simulink model "satcomv2"  (R2024b)
settings: Solver=VariableStepAuto  StartTime=0.0  StopTime=10.0  RelTol=1e-3
settings Model: Creator=user  LastModifiedBy=user

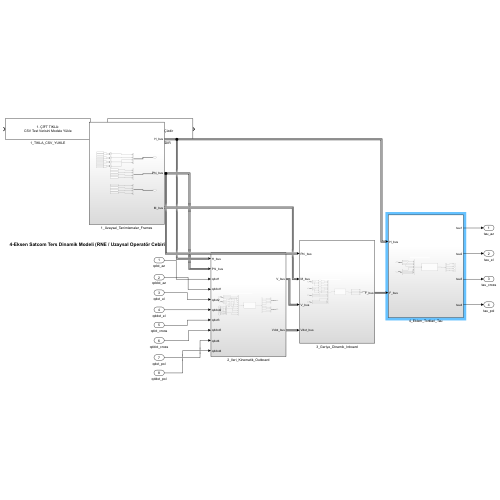
[thumbnail: Simulink's stored preview of the top-level diagram]
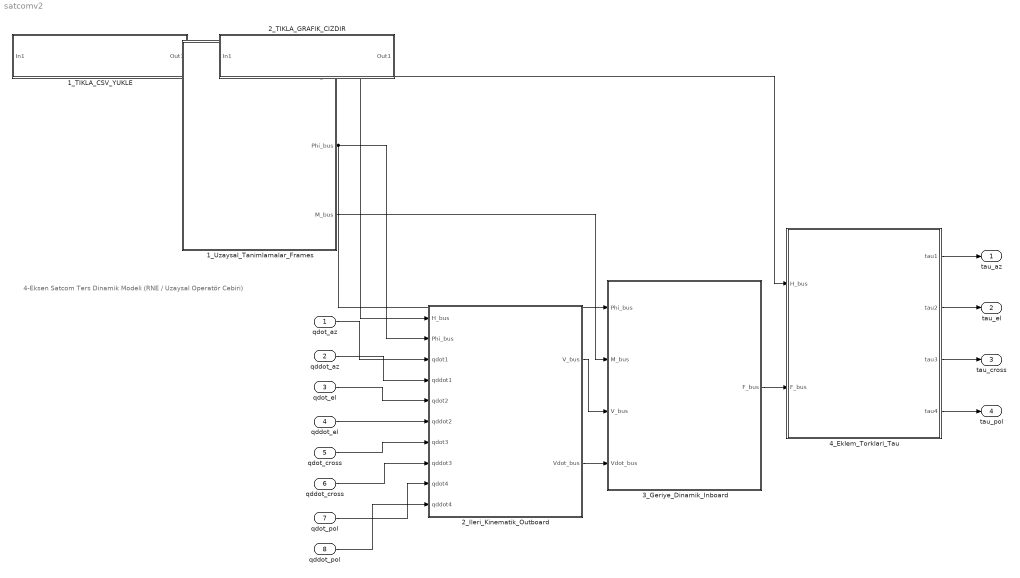
== system satcomv2 ==
  note: 4-Eksen Satcom Ters Dinamik Modeli (RNE / Uzaysal Operatör Cebiri)
  qdot_az : Inport
  qddot_az : Inport  Port=2
  qdot_el : Inport  Port=3
  qddot_el : Inport  Port=4
  qdot_cross : Inport  Port=5
  qddot_cross : Inport  Port=6
  qdot_pol : Inport  Port=7
  qddot_pol : Inport  Port=8
  1_TIKLA_CSV_YUKLE : Subsystem
      settings: OpenFcn=[f,p]=uigetfile({'*.csv;*.xlsx'}); if f~=0, mat=readmatrix(fullfile(p,f)); t=mat(:,2); t=t(:); v=mat(:,5); v=v(:); a=mat(:,7); a=a(:); % Sürücüden gelen akım (veya count) bilgisini Kt sabiti ile % çarparak motorun ürettiği gerçek Torka (Nm) dönüştürüyoruz.tau_real=mat(:,9) * 1.41; tau_real=tau_real(:); z=zeros(size(t)); assignin('base','in_qdot_az',timeseries(v,t)); assignin('base','in_qddot_az',timeseries(a,t)); assignin('base','in_zero',timeseries(z,t)); assignin('base','csv_zaman',t); assignin('base','csv_tork',tau_real); set_param(bdroot,'LoadExternalInput','on'); set_param(bdroot,'ExternalInput','in_qdot_az, in_qddot_az, in_zero, in_zero, in_zero, in_zero, in_zero, in_zero'); set_param(bdroot,'StopTime',num2str(t(end))); msgbox('Test Verileri Yüklendi! Sürücü çıkışı Kt=1.41 sabitiyle Nm cinsine dönüştürüldü.','BAŞARILI'); end
      mask Display: disp('1. ÇİFT TIKLA:\nCSV Test Verisini Modele Yükle');
  1_Uzaysal_Tanimlamalar_Frames : Subsystem
  2_Ileri_Kinematik_Outboard : Subsystem
  2_TIKLA_GRAFIK_CIZDIR : Subsystem
      settings: OpenFcn=try, simOut = evalin('base', 'out'); tau_raw = double(simOut.yout{1}.Values.Data(:)); t_sim = double(simOut.yout{1}.Values.Time(:)); [t_u, idx] = unique(t_sim); tau_u = tau_raw(idx); zaman = evalin('base', 'csv_zaman'); zaman = zaman(:); tau_real = evalin('base', 'csv_tork'); tau_real = tau_real(:); tau_model = interp1(t_u, tau_u, zaman, 'linear', 'extrap'); tau_model = tau_model(:); figure('Name', 'Saf Dinamik Model vs Gerçek Test', 'NumberTitle', 'off'); plot(zaman, tau_model, 'b', 'LineWidth', 1.5); hold on; plot(zaman, tau_real, 'r--', 'LineWidth', 1.2); title('Azimut Motoru - Tork İhtiyacı (Fiziksel Model vs Sürücü Çıkışı)'); xlabel('Zaman (s)'); ylabel('Tork (Nm)'); legend('Model Üretilen Tork (RNE İdeal Fiziği)', 'CSV İçindeki Gerçek Tork (Kt=1.41)'); grid on; SonucTablosu = table(zaman, tau_model, tau_real, 'VariableNames', {'Zaman_saniye', 'Model_Uretilen_Tork_Nm', 'Gercek_Sistem_Tork_Referansi'}); writetable(SonucTablosu, 'Model_Tork_Sonuclari.csv'); disp('Doğrulama verileri Model_Tork_Sonuclari.csv olarak başarıyla kaydedildi!'); catch ME, errordlg(sprintf('GRAFİK ÇİZİLEMEDİ!\\n\\nHata:\\n%s\\n\\nLütfen simülasyonu çalıştırdığınızdan (RUN) emin olun.', ME.message), 'Sistem Hatası'); end
      mask Display: disp('2. ÇİFT TIKLA:\nSaf Model Tork Grafiğini Çizdir');
  3_Geriye_Dinamik_Inboard : Subsystem
  4_Eklem_Torklari_Tau : Subsystem
  tau_az : Outport
  tau_el : Outport  Port=2
  tau_cross : Outport  Port=3
  tau_pol : Outport  Port=4
  wires:
  qddot_az/1 -> 2_Ileri_Kinematik_Outboard/4(qddot1)
  1_Uzaysal_Tanimlamalar_Frames/1(H_bus) -> 4_Eklem_Torklari_Tau/1(H_bus), 2_Ileri_Kinematik_Outboard/1(H_bus)
  1_Uzaysal_Tanimlamalar_Frames/2(Phi_bus) -> 3_Geriye_Dinamik_Inboard/1(Phi_bus), 2_Ileri_Kinematik_Outboard/2(Phi_bus)
  1_Uzaysal_Tanimlamalar_Frames/3(M_bus) -> 3_Geriye_Dinamik_Inboard/2(M_bus)
  qdot_az/1 -> 2_Ileri_Kinematik_Outboard/3(qdot1)
  qdot_el/1 -> 2_Ileri_Kinematik_Outboard/5(qdot2)
  qddot_el/1 -> 2_Ileri_Kinematik_Outboard/6(qddot2)
  qdot_cross/1 -> 2_Ileri_Kinematik_Outboard/7(qdot3)
  qddot_cross/1 -> 2_Ileri_Kinematik_Outboard/8(qddot3)
  qdot_pol/1 -> 2_Ileri_Kinematik_Outboard/9(qdot4)
  qddot_pol/1 -> 2_Ileri_Kinematik_Outboard/10(qddot4)
  2_Ileri_Kinematik_Outboard/1(V_bus) -> 3_Geriye_Dinamik_Inboard/3(V_bus)
  2_Ileri_Kinematik_Outboard/2(Vdot_bus) -> 3_Geriye_Dinamik_Inboard/4(Vdot_bus)
  3_Geriye_Dinamik_Inboard/1(F_bus) -> 4_Eklem_Torklari_Tau/2(F_bus)
  4_Eklem_Torklari_Tau/1(tau1) -> tau_az/1
  4_Eklem_Torklari_Tau/2(tau2) -> tau_el/1
  4_Eklem_Torklari_Tau/3(tau3) -> tau_cross/1
  4_Eklem_Torklari_Tau/4(tau4) -> tau_pol/1

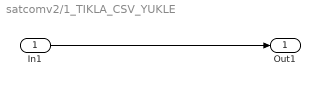
== system satcomv2/1_TIKLA_CSV_YUKLE ==
  In1 : Inport
  Out1 : Outport
  wires:
  In1/1 -> Out1/1

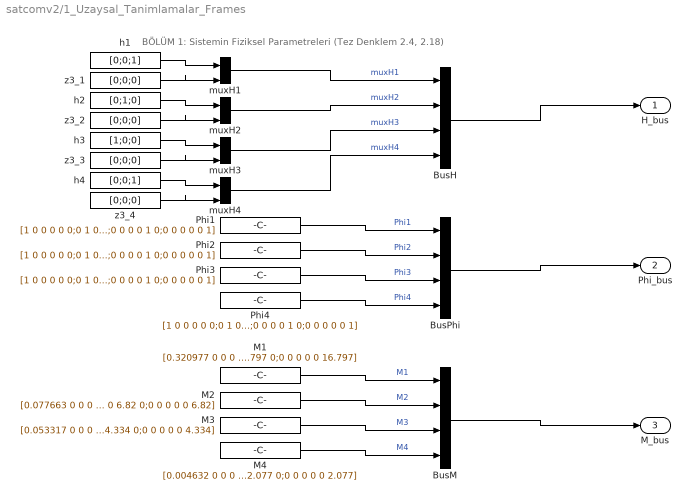
== system satcomv2/1_Uzaysal_Tanimlamalar_Frames ==
  note: BÖLÜM 1: Sistemin Fiziksel Parametreleri (Tez Denklem 2.4, 2.18)
  BusH : BusCreator  Inputs=4
  BusM : BusCreator  Inputs=4
  BusPhi : BusCreator  Inputs=4
  M1 : Constant  Value=[0.320977 0 0 0 0 0;0 0.320977 0 0 0 0;0 0 0.320977 0 0 0;0 0 0 16.797 0 0;0 0 0 0 16.797 0;0 0 0 0 0 16.797]
  M2 : Constant  Value=[0.077663 0 0 0 0 0;0 0.077663 0 0 0 0;0 0 0.077663 0 0 0;0 0 0 6.82 0 0;0 0 0 0 6.82 0;0 0 0 0 0 6.82]
  M3 : Constant  Value=[0.053317 0 0 0 0 0;0 0.053317 0 0 0 0;0 0 0.053317 0 0 0;0 0 0 4.334 0 0;0 0 0 0 4.334 0;0 0 0 0 0 4.334]
  M4 : Constant  Value=[0.004632 0 0 0 0 0;0 0.004632 0 0 0 0;0 0 0.004632 0 0 0;0 0 0 2.077 0 0;0 0 0 0 2.077 0;0 0 0 0 0 2.077]
  Phi{1..4} (4 alike) : Constant  Value=[1 0 0 0 0 0;0 1 0 0 0 0;0 0 1 0 0 0;0 0 0 1 0 0;0 0 0 0 1 0;0 0 0 0 0 1]
  h1 : Constant  Value=[0;0;1]
  h2 : Constant  Value=[0;1;0]
  h3 : Constant  Value=[1;0;0]
  h4 : Constant  Value=[0;0;1]
  muxH{1..4} (4 alike) : Mux  Inputs=2
  z3_{1..4} (4 alike) : Constant  Value=[0;0;0]
  H_bus : Outport
  Phi_bus : Outport  Port=2
  M_bus : Outport  Port=3
  wires:
  h1/1 -> muxH1/1
  z3_1/1 -> muxH1/2
  muxH1/1 -> BusH/1  "muxH1"
  h2/1 -> muxH2/1
  z3_2/1 -> muxH2/2
  muxH2/1 -> BusH/2  "muxH2"
  h3/1 -> muxH3/1
  z3_3/1 -> muxH3/2
  muxH3/1 -> BusH/3  "muxH3"
  h4/1 -> muxH4/1
  z3_4/1 -> muxH4/2
  muxH4/1 -> BusH/4  "muxH4"
  BusH/1 -> H_bus/1
  Phi1/1 -> BusPhi/1  "Phi1"
  Phi2/1 -> BusPhi/2  "Phi2"
  Phi3/1 -> BusPhi/3  "Phi3"
  Phi4/1 -> BusPhi/4  "Phi4"
  BusPhi/1 -> Phi_bus/1
  M1/1 -> BusM/1  "M1"
  M2/1 -> BusM/2  "M2"
  M3/1 -> BusM/3  "M3"
  M4/1 -> BusM/4  "M4"
  BusM/1 -> M_bus/1

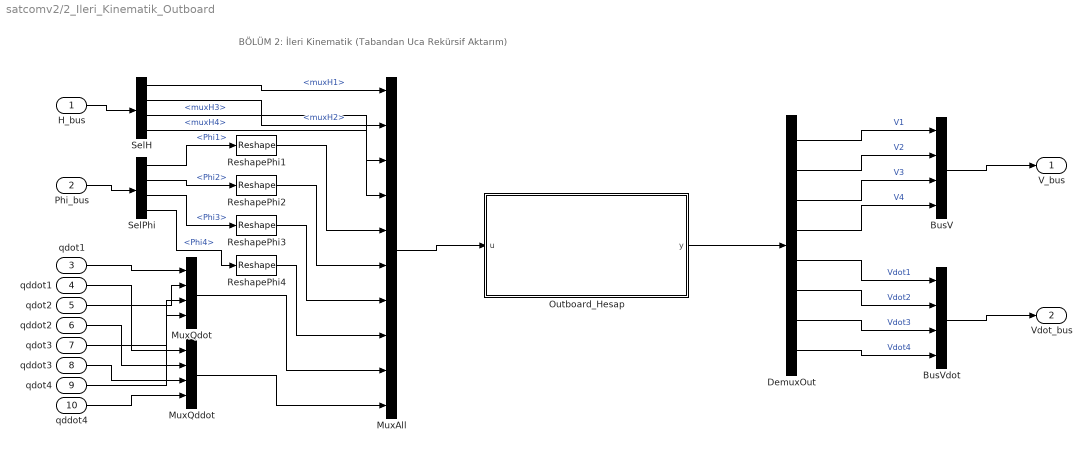
== system satcomv2/2_Ileri_Kinematik_Outboard ==
  note: BÖLÜM 2: İleri Kinematik (Tabandan Uca Rekürsif Aktarım)
  H_bus : Inport
  Phi_bus : Inport  Port=2
  qdot1 : Inport  Port=3
  qddot1 : Inport  Port=4
  qdot2 : Inport  Port=5
  qddot2 : Inport  Port=6
  qdot3 : Inport  Port=7
  qddot3 : Inport  Port=8
  qdot4 : Inport  Port=9
  qddot4 : Inport  Port=10
  BusV : BusCreator  Inputs=4
  BusVdot : BusCreator  Inputs=4
  DemuxOut : Demux  Outputs=[6 6 6 6 6 6 6 6]
  MuxAll : Mux  Inputs=10
  MuxQddot : Mux
  MuxQdot : Mux
  Outboard_Hesap : MATLAB Function  TreatAsAtomicUnit=on
  ReshapePhi{1..4} (4 alike) : Reshape
  SelH : BusSelector  OutputSignals=muxH1,muxH2,muxH3,muxH4
  SelPhi : BusSelector  OutputSignals=Phi1,Phi2,Phi3,Phi4
  V_bus : Outport
  Vdot_bus : Outport  Port=2
  wires:
  H_bus/1 -> SelH/1
  Phi_bus/1 -> SelPhi/1
  qdot1/1 -> MuxQdot/1
  qddot1/1 -> MuxQddot/1
  qdot2/1 -> MuxQdot/2
  qddot2/1 -> MuxQddot/2
  qdot3/1 -> MuxQdot/3
  qddot3/1 -> MuxQddot/3
  qdot4/1 -> MuxQdot/4
  qddot4/1 -> MuxQddot/4
  SelH/1 -> MuxAll/1  "<muxH1>"
  SelPhi/1 -> ReshapePhi1/1  "<Phi1>"
  ReshapePhi1/1 -> MuxAll/5
  SelH/2 -> MuxAll/2  "<muxH2>"
  SelPhi/2 -> ReshapePhi2/1  "<Phi2>"
  ReshapePhi2/1 -> MuxAll/6
  SelH/3 -> MuxAll/3  "<muxH3>"
  SelPhi/3 -> ReshapePhi3/1  "<Phi3>"
  ReshapePhi3/1 -> MuxAll/7
  SelH/4 -> MuxAll/4  "<muxH4>"
  SelPhi/4 -> ReshapePhi4/1  "<Phi4>"
  ReshapePhi4/1 -> MuxAll/8
  MuxQdot/1 -> MuxAll/9
  MuxQddot/1 -> MuxAll/10
  MuxAll/1 -> Outboard_Hesap/1(u)
  Outboard_Hesap/1(y) -> DemuxOut/1
  DemuxOut/1 -> BusV/1  "V1"
  DemuxOut/5 -> BusVdot/1  "Vdot1"
  DemuxOut/2 -> BusV/2  "V2"
  DemuxOut/6 -> BusVdot/2  "Vdot2"
  DemuxOut/3 -> BusV/3  "V3"
  DemuxOut/7 -> BusVdot/3  "Vdot3"
  DemuxOut/4 -> BusV/4  "V4"
  DemuxOut/8 -> BusVdot/4  "Vdot4"
  BusV/1 -> V_bus/1
  BusVdot/1 -> Vdot_bus/1

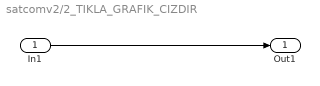
== system satcomv2/2_TIKLA_GRAFIK_CIZDIR ==
  In1 : Inport
  Out1 : Outport
  wires:
  In1/1 -> Out1/1

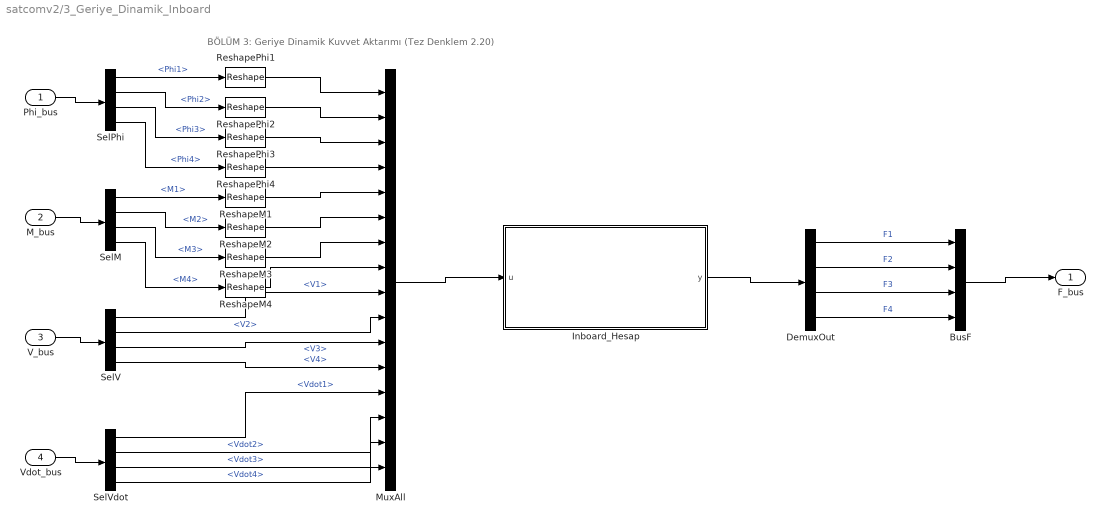
== system satcomv2/3_Geriye_Dinamik_Inboard ==
  note: BÖLÜM 3: Geriye Dinamik Kuvvet Aktarımı (Tez Denklem 2.20)
  Phi_bus : Inport
  M_bus : Inport  Port=2
  V_bus : Inport  Port=3
  Vdot_bus : Inport  Port=4
  BusF : BusCreator  Inputs=4
  DemuxOut : Demux  Outputs=[6 6 6 6]
  Inboard_Hesap : MATLAB Function  TreatAsAtomicUnit=on
  MuxAll : Mux  Inputs=16
  ReshapeM{1..4} (4 alike) : Reshape
  ReshapePhi{1..4} (4 alike) : Reshape
  SelM : BusSelector  OutputSignals=M1,M2,M3,M4
  SelPhi : BusSelector  OutputSignals=Phi1,Phi2,Phi3,Phi4
  SelV : BusSelector  OutputSignals=V1,V2,V3,V4
  SelVdot : BusSelector  OutputSignals=Vdot1,Vdot2,Vdot3,Vdot4
  F_bus : Outport
  wires:
  Phi_bus/1 -> SelPhi/1
  M_bus/1 -> SelM/1
  V_bus/1 -> SelV/1
  Vdot_bus/1 -> SelVdot/1
  SelPhi/1 -> ReshapePhi1/1  "<Phi1>"
  ReshapePhi1/1 -> MuxAll/1
  SelM/1 -> ReshapeM1/1  "<M1>"
  ReshapeM1/1 -> MuxAll/5
  SelV/1 -> MuxAll/9  "<V1>"
  SelVdot/1 -> MuxAll/13  "<Vdot1>"
  SelPhi/2 -> ReshapePhi2/1  "<Phi2>"
  ReshapePhi2/1 -> MuxAll/2
  SelM/2 -> ReshapeM2/1  "<M2>"
  ReshapeM2/1 -> MuxAll/6
  SelV/2 -> MuxAll/10  "<V2>"
  SelVdot/2 -> MuxAll/14  "<Vdot2>"
  SelPhi/3 -> ReshapePhi3/1  "<Phi3>"
  ReshapePhi3/1 -> MuxAll/3
  SelM/3 -> ReshapeM3/1  "<M3>"
  ReshapeM3/1 -> MuxAll/7
  SelV/3 -> MuxAll/11  "<V3>"
  SelVdot/3 -> MuxAll/15  "<Vdot3>"
  SelPhi/4 -> ReshapePhi4/1  "<Phi4>"
  ReshapePhi4/1 -> MuxAll/4
  SelM/4 -> ReshapeM4/1  "<M4>"
  ReshapeM4/1 -> MuxAll/8
  SelV/4 -> MuxAll/12  "<V4>"
  SelVdot/4 -> MuxAll/16  "<Vdot4>"
  MuxAll/1 -> Inboard_Hesap/1(u)
  Inboard_Hesap/1(y) -> DemuxOut/1
  DemuxOut/1 -> BusF/1  "F1"
  DemuxOut/2 -> BusF/2  "F2"
  DemuxOut/3 -> BusF/3  "F3"
  DemuxOut/4 -> BusF/4  "F4"
  BusF/1 -> F_bus/1

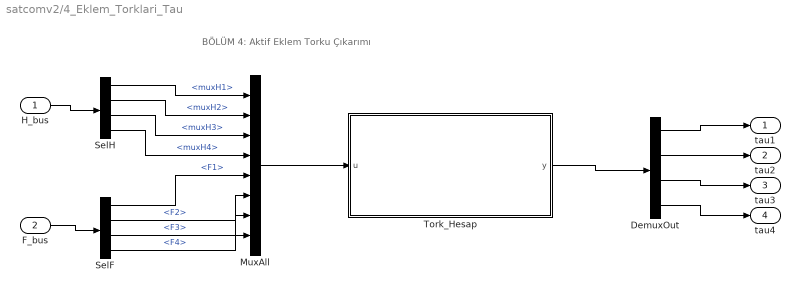
== system satcomv2/4_Eklem_Torklari_Tau ==
  note: BÖLÜM 4: Aktif Eklem Torku Çıkarımı
  H_bus : Inport
  F_bus : Inport  Port=2
  DemuxOut : Demux  Outputs=[1 1 1 1]
  MuxAll : Mux  Inputs=8
  SelF : BusSelector  OutputSignals=F1,F2,F3,F4
  SelH : BusSelector  OutputSignals=muxH1,muxH2,muxH3,muxH4
  Tork_Hesap : MATLAB Function  TreatAsAtomicUnit=on
  tau1 : Outport
  tau2 : Outport  Port=2
  tau3 : Outport  Port=3
  tau4 : Outport  Port=4
  wires:
  H_bus/1 -> SelH/1
  F_bus/1 -> SelF/1
  SelH/1 -> MuxAll/1  "<muxH1>"
  SelF/1 -> MuxAll/5  "<F1>"
  SelH/2 -> MuxAll/2  "<muxH2>"
  SelF/2 -> MuxAll/6  "<F2>"
  SelH/3 -> MuxAll/3  "<muxH3>"
  SelF/3 -> MuxAll/7  "<F3>"
  SelH/4 -> MuxAll/4  "<muxH4>"
  SelF/4 -> MuxAll/8  "<F4>"
  MuxAll/1 -> Tork_Hesap/1(u)
  Tork_Hesap/1(y) -> DemuxOut/1
  DemuxOut/1 -> tau1/1
  DemuxOut/2 -> tau2/1
  DemuxOut/3 -> tau3/1
  DemuxOut/4 -> tau4/1

== matlab function satcomv2/2_Ileri_Kinematik_Outboard/Outboard_Hesap ==
  data: u input; y output
function y = fcn(u)
% =========================================================================
% İLERİ KİNEMATİK (OUTBOARD PROPAGATION / FORWARD KINEMATICS)
% Referans: S. Murat Yeşiloğlu (2007) Ph.D. Thesis, Bölüm 2.
%
% Açıklama: Bu fonksiyon, tabandan (base) uca (tip) doğru ilerleyerek
% her bir uzvun uzaysal hız (V) ve uzaysal ivmelerini (Vdot) hesaplar.
% Üst uzvun hızı, alt uzvun taşıma hızı ile kendi rölatif hızının toplamıdır.
% =========================================================================

% --- 1. HAFIZA TAHSİSİ VE GİRİŞ (u) PARÇALAMA ---
H = cell(4,1);   % Eklem Hareket Ekseni Vektörleri (6x1)
Phi = cell(4,1); % Uzaysal Dönüşüm / Geçiş Matrisleri (6x6)
idx = 1;

% u vektöründen 6x1'lik H (Eksen) vektörleri çekilir (24 eleman)
for k=1:4, H{k} = u(idx:idx+5); idx = idx + 6; end

% u vektöründen 6x6'lık Phi (Geometri/Geçiş) matrisleri çekilir (144 eleman)
for k=1:4, Phi{k} = reshape(u(idx:idx+35), 6, 6); idx = idx + 36; end

% u vektöründen skaler q_dot (Eklem açısal hızları) çekilir (4 eleman)
qdot = u(idx:idx+3); idx = idx + 4; 

% u vektöründen skaler q_ddot (Eklem açısal ivmeleri) çekilir (4 eleman)
qddot = u(idx:idx+3);

% --- 2. BAŞLANGIÇ KOŞULLARI (BASE CONDITIONS) ---
% Taban (Base) yere sabitlendiği için ilk hız ve ivme SIFIR kabul edilir.
% Eğer sistem hareketli bir araç (gemi/uçak) üzerinde olsaydı, buraya 
% aracın hız ve ivme (roll, pitch, yaw vb.) değerleri girilirdi.
Vprev = zeros(6,1);    % V_0 = 0
Vdotprev = zeros(6,1); % Vdot_0 = 0

V = cell(4,1);  % Hesaplanacak uzaysal hızları tutacak bellek
Vd = cell(4,1); % Hesaplanacak uzaysal ivmeleri tutacak bellek


% --- 3. İLERİYE DOĞRU (BASE -> TIP) HIZ VE İVME AKTARIMI ---
for k=1:4
  % TEZ DENKLEM (2.3) VE (2.8): UZAYSAL HIZ AKTARIMI
  % V_k = Phi_{k,k-1} * V_{k-1} + H_k * qdot_k
  % Fiziksel Anlamı: k. uzvun hızı = (Bir önceki uzvun bu uzva taşınan hızı) + (Motorun kendi dönme hızı)
  Vk  = Phi{k} * Vprev + H{k} * qdot(k);
  
  % TEZ DENKLEM (2.13) VE (2.16): UZAYSAL İVME AKTARIMI
  % Vdot_k = Phi_{k,k-1} * Vdot_{k-1} + H_k * qddot_k + (V_k X (H_k * qdot_k))
  % Fiziksel Anlamı: 
  % 1. Terim (Phi*Vdotprev) : Bir önceki uzvun taşıma ivmesi.
  % 2. Terim (H*qddot)      : Motorun kendi saf ivmelenmesi.
  % 3. Terim (crm(Vk)...)   : Dönen bir sistemde oluşan Jiroskopik / Coriolis hızlanmasıdır.
  Vdk = Phi{k} * Vdotprev + H{k} * qddot(k) + crm(Vk) * (H{k} * qdot(k));
  
  % Hesaplanmış bu değerleri kaydet ve bir sonraki döngü için 'prev' yap
  V{k} = Vk; 
  Vd{k} = Vdk; 
  
  Vprev = Vk; 
  Vdotprev = Vdk;
end

% --- 4. ÇIKIŞ (y) VEKTÖRÜNÜ HAZIRLAMA ---
y = zeros(48,1); % 4x6 (Hızlar) + 4x6 (İvmeler) = Toplam 48 elemanlık çıkış
idx = 1;

% Bütün hızları y vektörünün ilk yarısına diz
for k=1:4, y(idx:idx+5) = V{k}; idx = idx + 6; end

% Bütün ivmeleri y vektörünün ikinci yarısına diz
for k=1:4, y(idx:idx+5) = Vd{k}; idx = idx + 6; end

end

% =========================================================================
% =========================================================================

% Hareket için Vektörel Çarpım (Spatial Cross Product for Motion)
% 6 boyutlu bir hız vektörünü V=[w; v], diğer bir hareket vektörüyle (örn: H*qdot) 
% vektörel olarak çarpmak için 6x6'lık matris formuna dönüştürür.
function X=crm(V)
    w = V(1:3); % Açısal hız (omega)
    v = V(4:6); % Çizgisel hız (velocity)
    X = [skew(w), zeros(3,3); 
         skew(v), skew(w)]; 
end

% Anti-Simetrik Matris (Skew-Symmetric Matrix)
% Klasik 3D a x b vektörel çarpımını, matris çarpımı [a_skew]*b yapmak için kullanılır.
function S=skew(a)
    S = [ 0,    -a(3),  a(2); 
          a(3),  0,    -a(1); 
         -a(2),  a(1),  0   ]; 
end

== matlab function satcomv2/4_Eklem_Torklari_Tau/Tork_Hesap ==
  data: u input; y output
function y = fcn(u)
% =========================================================================
% AKTİF EKLEM TORKU İZDÜŞÜMÜ (JOINT TORQUE PROJECTION)
% Referans: S. Murat Yeşiloğlu (2007) Ph.D. Thesis, Bölüm 2.
%
% Açıklama: Bu fonksiyon, Inboard aşamasında hesaplanan 6 boyutlu uzaysal 
% kuvvet/moment yığınının (F) içinden, sadece motorun kendi dönme eksenindeki 
% (H) 1 boyutlu (skaler) tork ihtiyacını (tau) çekip çıkarma işlemini yapar.
% =========================================================================

% --- 1. HAFIZA TAHSİSİ VE GİRİŞ (u) PARÇALAMA ---
H = cell(4,1); % Eklem Hareket Ekseni (Serbestlik) Vektörleri (6x1)
F = cell(4,1); % Ekleme Binen Toplam Uzaysal Kuvvetler (6x1)
idx = 1;

% u vektörünün ilk 24 elemanından 6x1 boyutundaki H vektörleri çekilir.
% H vektörü, motorun sadece hangi yönde serbestçe döndüğünü (örneğin sadece 
% Z ekseni etrafında) belirten uzaysal bir filtredir.
for k=1:4
    H{k} = u(idx:idx+5); 
    idx = idx + 6; 
end

% u vektörünün kalan 24 elemanından 6x1 boyutundaki F vektörleri çekilir.
% F = [Mx; My; Mz; fx; fy; fz] formundadır ve sistemin tüm yanal ezilme, 
% bükülme ve dönme yüklerini aynı anda barındırır.
for k=1:4
    F{k} = u(idx:idx+5); 
    idx = idx + 6; 
end

% --- 2. İZDÜŞÜM (PROJECTION) VE TORK HESAPLAMASI ---
y = zeros(4,1); % 4 motorun üreteceği skaler tork (Nm) çıkış vektörü

for k=1:4
    % DENKLEM: tau_k = H_k^T * F_k
    % Transpoz (H') alma işlemi, iki uzaysal vektörün iç çarpımını (dot product) yapar.
    % Fiziksel Anlamı: Matris çarpımı sayesinde, motorun dönmediği 5 eksendeki 
    % (X, Y bükülmeleri ve X, Y, Z itmeleri) tüm yükler sıfırla çarpılarak yutulur. 
    % Çünkü o yükleri motor değil, makinenin şasesi ve rulmanları taşır.
    % Geriye kalan tek değer, sürücünün motora basması gereken saf torktur.
    
    y(k) = H{k}' * F{k}; 
end

end

== matlab function satcomv2/3_Geriye_Dinamik_Inboard/Inboard_Hesap ==
  data: u input; y output
function y = fcn(u)
% =========================================================================
% GERİYE DOĞRU DİNAMİK KUVVET AKTARIMI (INBOARD FORCE RECURSION)
% Referans: S. Murat Yeşiloğlu (2007) Ph.D. Thesis, Bölüm 2.
%
% Bu fonksiyon, Outboard aşamasında hesaplanan uzaysal hız (V) ve 
% ivmeleri (Vd) kullanarak, en uç noktadan (tip) tabana (base) doğru 
% uzaysal kuvvetleri (F) hesaplar ve alt uzuvlara aktarır.
% =========================================================================

% --- 1. HAFIZA (CELL ARRAY) TANIMLAMALARI VE GİRİŞ (u) PARÇALAMA ---
Phi = cell(4,1);   % Uzaysal Dönüşüm (Geometri/Geçiş) Matrisleri (6x6)
I_mat = cell(4,1); % Uzaysal Atalet Matrisleri (Kütle ve Eylemsizlik) (6x6)
V = cell(4,1);     % Uzaysal Hız Vektörleri (6x1)
Vd = cell(4,1);    % Uzaysal İvme Vektörleri (6x1)
idx = 1;           % Tek boyutlu 'u' vektöründen okuma yapmak için indeks

% u vektöründen 6x6'lık Phi (Geometri) matrisleri çekiliyor (144 eleman)
for k=1:4, Phi{k} = reshape(u(idx:idx+35), 6, 6); idx = idx + 36; end

% u vektöründen 6x6'lık I_mat (Atalet) matrisleri çekiliyor (144 eleman)
for k=1:4, I_mat{k} = reshape(u(idx:idx+35), 6, 6); idx = idx + 36; end

% u vektöründen 6x1'lik V (Hız) vektörleri çekiliyor (24 eleman)
for k=1:4, V{k} = u(idx:idx+5); idx = idx + 6; end

% u vektöründen 6x1'lik Vdot (İvme) vektörleri çekiliyor (24 eleman)
for k=1:4, Vd{k} = u(idx:idx+5); idx = idx + 6; end


% --- 2. GERİYE DOĞRU (TIP -> BASE) NEWTON-EULER HESAPLAMASI ---
F = cell(4,1);         % Her eksende biriken toplam uzaysal kuvvet
Fchild = zeros(6,1);   % Üstteki (çocuk) uzuvdan gelen yük. En uçta boşluk olduğu için sıfırla başlar.

% Döngü 4'ten 1'e doğru (Uçtan Tabana) çalışır
for k=4:-1:1
    
    % DENKLEM (2.20): F_k = M_k * Vdot_k + b_k + F_child
    % Fk: k'ncı eklemin merkezine etki eden net kuvvet ve moment (Tork) ihtiyacıdır.
    % 1. Terim (I_mat{k}*Vd{k})       : Newton'un F = m*a'sı. Salt atalet kuvveti.
    % 2. Terim (crf(V)*(I_mat*V))     : Coriolis ve Merkezkaç (bias) kuvvetleri (b_k).
    % 3. Terim (Fchild)               : Kendisinden sonraki uzuvların yarattığı ağırlık ve dinamik yük.
    Fk = I_mat{k}*Vd{k} + crf(V{k})*(I_mat{k}*V{k}) + Fchild;
    
    % Hesaplanmış bu net kuvveti k. eksen için kaydet
    F{k} = Fk;
    
    % KUVVET AKTARIMI (FORCE PROPAGATION):
    % Eğer tabana (1. eksen) henüz gelmediysek, hesaplanan bu kuvveti 
    % bir alttaki eksenin kucağına (Fchild olarak) bırakmamız gerekir.
    % Kinematikte (Outboard) geçiş matrisi Phi iken, Fizikte (Inboard) dualite 
    % kuralı gereği Phi'nin transpozu (Phi') kullanılır.
    if k>1
        Fchild = Phi{k}' * Fk; 
    end
end

% --- 3. ÇIKIŞ (y) VEKTÖRÜNÜ HAZIRLAMA ---
y = zeros(24,1); 
idx = 1;
% 4 adet 6x1 boyutundaki kuvvet vektörünü, tek bir 24x1 sütun haline getirir
for k=1:4, y(idx:idx+5) = F{k}; idx = idx + 6; end
end

% =========================================================================
% YARDIMCI MATEMATİKSEL OPERATÖRLER (UZAYSAL CEBİR KÜTÜPHANESİ)

% (Spatial Cross Product for Forces)
% Hareket operatörünün negatif transpozudur.
function X=crf(V)
    X = -crm(V)'; 
end

% (Spatial Cross Product for Motion)
% 6 boyutlu bir hız vektörünü V=[w; v], 6x6 matris formuna dönüştürür.
function X=crm(V)
    w = V(1:3); % Açısal hız (omega)
    v = V(4:6); % Çizgisel hız (velocity)
    X = [skew(w), zeros(3,3); 
         skew(v), skew(w)]; 
end

% Klasik 3D a x b vektörel çarpımını, matris çarpımı [a_skew]*b yapmak için kullanılır.
function S=skew(a)
    S = [ 0,    -a(3),  a(2); 
          a(3),  0,    -a(1); 
         -a(2),  a(1),  0   ]; 
end
